simulink model "ccpitf"  (Simulink 7.9)
settings: Solver=ode45  SolverMode=SingleTasking  StartTime=0.0  StopTime=10  RelTol=1e-3  AbsTol=1e-6
undefined symbols (not defined in the file): b, Ki, Kp, m
settings Model: Creator=Rick  LastModifiedBy=Rick
settings DataIOCC: LimitDataPoints=off
settings OptimizationCC: BlockReduction=off  BooleanDataType=off
settings DebuggingCC: SaveWithParameterizedLinksMsg=none  SignalResolutionControl=TryResolveAllWithWarning  SolverPrmCheckMsg=none  MultiTaskDSMMsg=warning  MultiTaskCondExecSysMsg=none  StrictBusMsg=None
settings HardwareCC: TargetUnknown=on
settings RTWCC: IncludeERTFirstTime=on

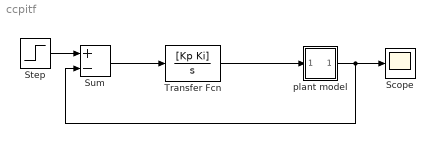
== system ccpitf ==
  Scope : Scope
      settings: TickLabels=on
  Step : Step  Time=0  After=10
  Sum : Sum  Inputs=+-  SaturateOnIntegerOverflow=on  InputSameDT=on  OutDataTypeStr=Inherit: Same as first input
  Transfer Fcn : TransferFcn  Numerator=[Kp Ki]  Denominator=[1 0]
  plant model : Subsystem
  wires:
  plant model/1(Out) -> Scope/1, Sum/2
  Transfer Fcn/1 -> plant model/1(In)
  Sum/1 -> Transfer Fcn/1
  Step/1 -> Sum/1

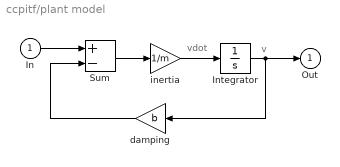
== system ccpitf/plant model ==
  note: v
  note: vdot
  In : Inport
  Integrator : Integrator
  Sum : Sum  Inputs=+-  SaturateOnIntegerOverflow=on  InputSameDT=on  OutDataTypeStr=Inherit: Same as first input
  damping : Gain  Gain=b  SaturateOnIntegerOverflow=on  OutDataTypeStr=Inherit: Same as input  ParamDataTypeStr=Inherit: Same as input
  inertia : Gain  Gain=1/m  SaturateOnIntegerOverflow=on  OutDataTypeStr=Inherit: Same as input  ParamDataTypeStr=Inherit: Same as input
  Out : Outport  InitialOutput=0
  wires:
  inertia/1 -> Integrator/1
  Sum/1 -> inertia/1
  damping/1 -> Sum/2
  Integrator/1 -> Out/1, damping/1
  In/1 -> Sum/1
